simulink model "HW1_b"  (R2025b)
settings: Solver=VariableStepAuto  StartTime=0.0  StopTime=10.0  RelTol=1e-3
values from neighbouring files (symbols this model uses):
  A = 8e-4    (= 0.0008)    [parameters.m]
  Bm = 1e-6    (= 1e-06)    [parameters.m]
  Jd = 1e-7    (= 1e-07)    [parameters.m]
  Jm = 10.8e-7    (= 1.08e-06)    [parameters.m]
  Kb = 0.0234    [parameters.m]
  Kd = 2.4    [parameters.m]
  Kp = 1e-6    (= 1e-06)    [parameters.m]
  Ks = 50    [parameters.m]
  Kt = 0.0234    [parameters.m]
  Kx = 1.17    [parameters.m]
  La = 0.238e-3    (= 0.000238)    [parameters.m]
  M = 15    [parameters.m]
  r = 0.0016    [parameters.m]
  Ra = 2.32    [parameters.m]
settings Model: Creator=hasan  LastModifiedBy=hasan

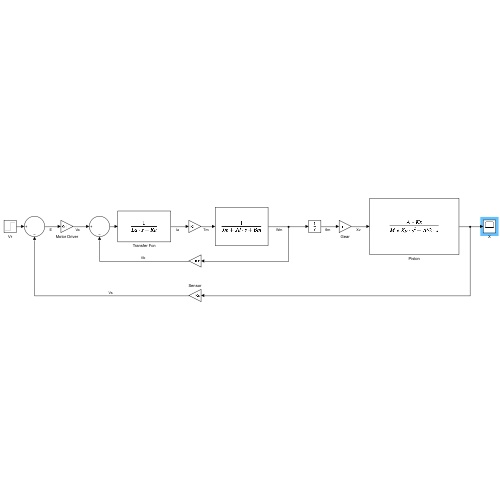
[thumbnail: Simulink's stored preview of the top-level diagram]
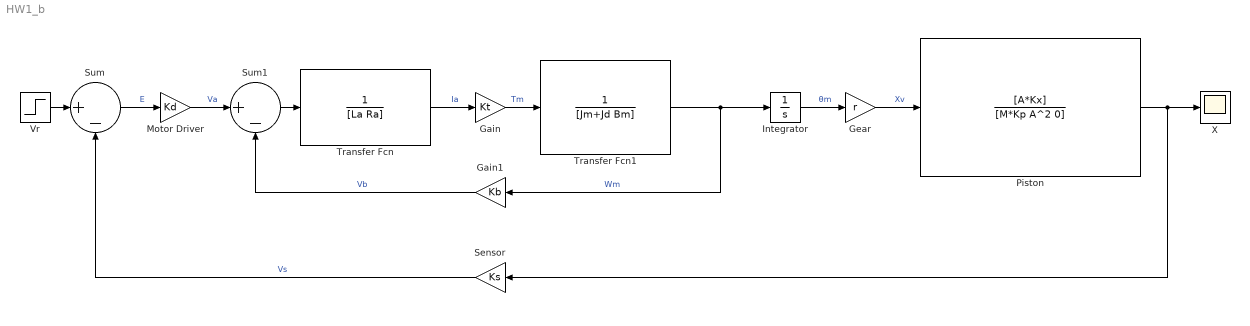
== system HW1_b ==
  Gain : Gain  Gain=Kt
  Gain1 : Gain  Gain=Kb
  Gear : Gain  Gain=r
  Integrator : Integrator
  Motor Driver : Gain  Gain=Kd
  Piston : TransferFcn  Numerator=[A*Kx]  Denominator=[M*Kp A^2 0]
  Sensor : Gain  Gain=Ks
  Sum : Sum  Inputs=|+-
  Sum1 : Sum  Inputs=|+-
  Transfer Fcn : TransferFcn  Denominator=[La Ra]
  Transfer Fcn1 : TransferFcn  Denominator=[Jm+Jd Bm]
  Vr : Step  SampleTime=0
  X : Scope
      settings: ActiveDisplayYMinimum=-5.3326753008335209E+8  ActiveDisplayYMaximum=9.2328609334516048E+8
  wires:
  Vr/1 -> Sum/1
  Sum/1 -> Motor Driver/1  "E"
  Sum1/1 -> Transfer Fcn/1
  Transfer Fcn/1 -> Gain/1  "Ia"
  Gain/1 -> Transfer Fcn1/1  "Tm"
  Transfer Fcn1/1 -> Gain1/1, Integrator/1  "Wm"
  Gain1/1 -> Sum1/2  "Vb"
  Integrator/1 -> Gear/1  "θm"
  Gear/1 -> Piston/1  "Xv"
  Piston/1 -> X/1, Sensor/1
  Sensor/1 -> Sum/2  "Vs"
  Motor Driver/1 -> Sum1/1  "Va"
